simulink model "sim_model"  (R2020a)
settings: Solver=VariableStepAuto  StartTime=0.0  StopTime=30  RelTol=1e-3
model workspace (MAT data in the model file):
  r = Simulink.Parameter
  r.Value = 1
  r.DataType = 'auto'
  r.Dimensions = [1 1]
settings Model: Creator=mvisc  LastModifiedBy=mvisc

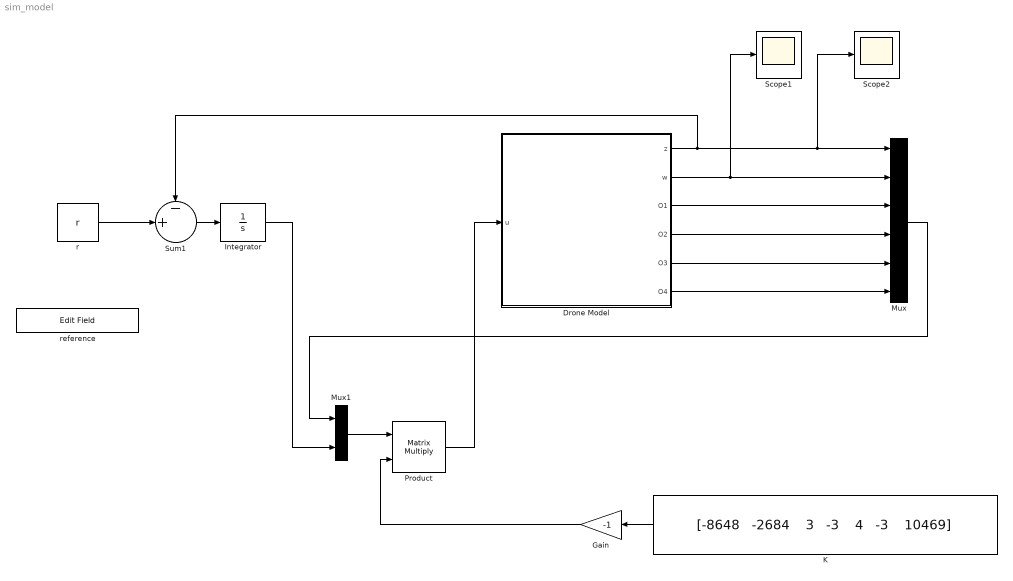
== system sim_model ==
  Drone Model : Subsystem
  Gain : Gain  Gain=-1
  Integrator : Integrator
  K : Constant  Value="[-8648   -2684    3   -3    4   -3    10469]"
  Mux : Mux  Inputs=6
  Mux1 : Mux  Inputs=2
  Product : Product  Multiplication=Matrix(*)
  Scope1 : Scope
  Scope2 : Scope
  Sum1 : Sum  Inputs=-+|
  r : Constant  Value=r
  reference : EditField  LabelPosition=Hide  ShowInitialText=on  Alignment=Center
  wires:
  Drone Model/1(z) -> Scope2/1, Mux/1, Sum1/1
  Drone Model/2(w) -> Mux/2, Scope1/1
  Product/1 -> Drone Model/1(u)
  Drone Model/3(O1) -> Mux/3
  Drone Model/4(O2) -> Mux/4
  Drone Model/5(O3) -> Mux/5
  Drone Model/6(O4) -> Mux/6
  K/1 -> Gain/1
  Gain/1 -> Product/2
  Sum1/1 -> Integrator/1
  Mux1/1 -> Product/1
  Mux/1 -> Mux1/1
  Integrator/1 -> Mux1/2
  r/1 -> Sum1/2

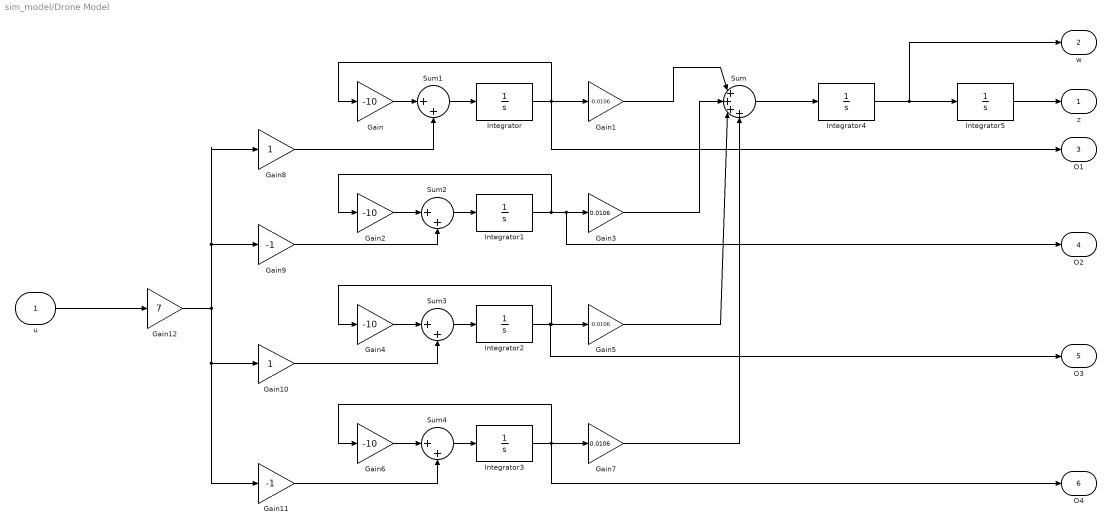
== system sim_model/Drone Model ==
  u : Inport
  Gain{,2,4,6} (4 alike) : Gain  Gain=-10
  Gain1 : Gain  Gain=-0.0106
  Gain10 : Gain
  Gain11 : Gain  Gain=-1
  Gain12 : Gain  Gain=7
  Gain3 : Gain  Gain=0.0106
  Gain5 : Gain  Gain=-0.0106
  Gain7 : Gain  Gain=0.0106
  Gain8 : Gain
  Gain9 : Gain  Gain=-1
  Integrator{,1..5} (6 alike) : Integrator
  Sum : Sum  Inputs=|++++
  Sum{1..4} (4 alike) : Sum  Inputs=|++
  z : Outport
  w : Outport  Port=2
  O1 : Outport  Port=3
  O2 : Outport  Port=4
  O3 : Outport  Port=5
  O4 : Outport  Port=6
  wires:
  Sum4/1 -> Integrator3/1
  Sum2/1 -> Integrator1/1
  Integrator/1 -> Gain1/1, O1/1, Gain/1
  Gain1/1 -> Sum/1
  Gain/1 -> Sum1/1
  Integrator2/1 -> O3/1, Gain5/1, Gain4/1
  Integrator1/1 -> O2/1, Gain3/1, Gain2/1
  Gain4/1 -> Sum3/1
  Gain3/1 -> Sum/2
  Sum3/1 -> Integrator2/1
  Gain2/1 -> Sum2/1
  Gain6/1 -> Sum4/1
  Integrator5/1 -> z/1
  Gain7/1 -> Sum/4
  Integrator3/1 -> Gain6/1, O4/1, Gain7/1
  Sum/1 -> Integrator4/1
  Sum1/1 -> Integrator/1
  Gain5/1 -> Sum/3
  Integrator4/1 -> w/1, Integrator5/1
  Gain8/1 -> Sum1/2
  Gain9/1 -> Sum2/2
  Gain10/1 -> Sum3/2
  Gain11/1 -> Sum4/2
  Gain12/1 -> Gain9/1, Gain8/1, Gain10/1, Gain11/1
  u/1 -> Gain12/1
